simulink model "NONLINEAR_MODEL11"  (R2017b)
settings: Solver=VariableStepAuto  StartTime=0.0  StopTime=50  RelTol=1e-3
values from neighbouring files (symbols this model uses):
  altitude = input('Enter the altitude for the simulation (ft)  :  ')    [FindF16Dynamics.m]    (also in run_me.m = input(' altitude ( 0 ~ 40000 ft ) : '); trim_F16.m = alt)
  control_trim = u0    [find_trim.m]
  state_trim = steady_state( state )    [find_trim.m]
  trim_state = xu(1:12)    [trim_F16.m]
  velocity = input('Enter the velocity for the simulation (ft/s):  ')    [FindF16Dynamics.m]    (also in run_me.m = input(' true velocity ( 350 ~ 1000 ft/sec ) : '); trim_F16.m = vel)
libraries: simulink x7, F16_Actuator_Library x1
settings Model: Creator=monster  LastModifiedBy=monster

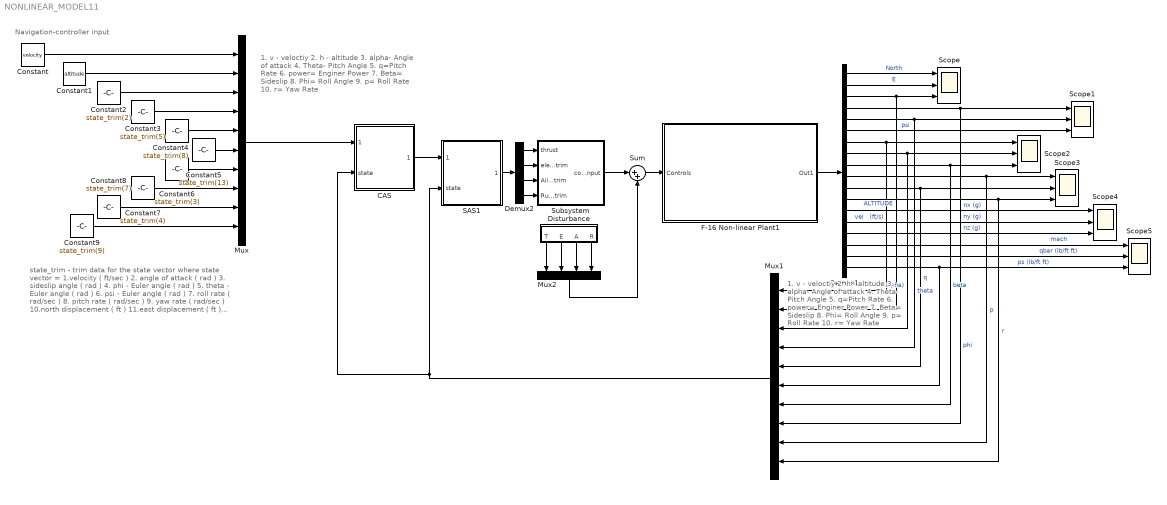
== system NONLINEAR_MODEL11 ==
  note: Navigation-controller input
  note: 1. v - veloctiy
      |
      | 2. h - altitude
      |
      | 3. alpha- Angle of attack
      |
      | 4. Theta- Pitch Angle
      |
      | 5. q=Pitch Rate
      |
      | 6. power= Enginer Power
      |
      | 7. Beta= Sideslip
      |
      | 8. Phi= Roll Angle
      |
      | 9. p= Roll Rate
      |
      | 10. r= Yaw Rate
  note: 1. v - veloctiy
      |
      | 2. h - altitude
      |
      | 3. alpha- Angle of attack
      |
      | 4. Theta- Pitch Angle
      |
      | 5. q=Pitch Rate
      |
      | 6. power= Enginer Power
      |
      | 7. Beta= Sideslip
      |
      | 8. Phi= Roll Angle
      |
      | 9. p= Roll Rate
      |
      | 10. r= Yaw Rate
  note: state_trim   - trim data for the state vector where
      |       state vector =
      | 1.velocity             ( ft/sec )
      | 2. angle of attack      ( rad )
      |  3. sideslip angle       ( rad )
      | 4. phi   - Euler angle  ( rad )
      | 5. theta - Euler angle  ( rad )
      |    6. psi   - Euler angle  ( rad )
      |   7. roll rate            ( rad/sec )
      | 8. pitch rate           ( rad/sec )
      |  9. yaw rate             ( rad/sec )
      | 10.north displacement   ( ft )
      | 11.east displacement    ( ft )
      | 12.altitude             ( ft )
      | 13.power  ( percent, 0 <= pow <= 100 )
  " Disturbance" : Subsystem
  CAS : Subsystem
  Constant : Constant  Value=velocity
  Constant1 : Constant  Value=altitude
  Constant2 : Constant  Value=state_trim(2)
  Constant3 : Constant  Value=state_trim(5)
  Constant4 : Constant  Value=state_trim(8)
  Constant5 : Constant  Value=state_trim(13)
  Constant6 : Constant  Value=state_trim(3)
  Constant7 : Constant  Value=state_trim(4)
  Constant8 : Constant  Value=state_trim(7)
  Constant9 : Constant  Value=state_trim(9)
  Demux1 : Demux  Outputs=18
  Demux2 : Demux
  F-16 Non-linear Plant1 : Subsystem
      mask Display: image('D:\Dropbox\M.eng\fall2017\flight control system\FDC\project\control surface.PNG');
  Mux : Mux  Inputs=10
  Mux1 : Mux  Inputs=10
  Mux2 : Mux
  SAS1 : Subsystem
  Scope{,1..5} (6 alike) : Scope  NumInputPorts=3
  Subsystem : Subsystem
  Sum : Sum  Inputs=|++
  wires:
  Demux1/11 -> Scope3/2, Mux1/5  "q"
  Demux1/18 -> Mux1/6, Scope5/3  "ps (lb/ft ft)"
  Demux1/16 -> Scope5/1  "mach"
  Demux1/17 -> Scope5/2  "qbar (lb/ft ft)"
  F-16 Non-linear Plant1/1(Out1) -> Demux1/1
  Demux1/7 -> Mux1/1, Scope2/1  "vel   (ft/s)"
  Demux1/10 -> Mux1/9, Scope3/1  "p"
  Demux1/9 -> Mux1/7, Scope2/3  "beta"
  Demux1/6 -> Scope1/3  "psi"
  Demux1/14 -> Scope4/2  "ny (g)"
  Demux1/2 -> Scope/2  "E"
  Demux1/12 -> Mux1/10, Scope3/3  "r"
  Demux1/5 -> Mux1/4, Scope1/2  "theta"
  Demux1/15 -> Scope4/3  "nz (g)"
  Demux1/3 -> Mux1/2, Scope/3  "ALTITUDE"
  Demux1/1 -> Scope/1  "North"
  Demux1/8 -> Mux1/3, Scope2/2  "alpha)"
  Demux1/4 -> Mux1/8, Scope1/1  "phi"
  Demux1/13 -> Scope4/1  "nx (g)"
  Constant4/1 -> Mux/5
  " Disturbance"/1(T) -> Mux2/1
  Mux2/1 -> Sum/2
  Constant2/1 -> Mux/3
  Mux1/1 -> CAS/2(state), SAS1/2(state)
  Constant7/1 -> Mux/8
  Constant9/1 -> Mux/10
  Mux/1 -> CAS/1(reference)
  SAS1/1(control_input) -> Demux2/1
  Demux2/4 -> Subsystem/4(Rudder_trim)
  Constant5/1 -> Mux/6
  Constant8/1 -> Mux/9
  Subsystem/1(control_input) -> Sum/1
  Demux2/1 -> Subsystem/1(thrust)
  " Disturbance"/4(R) -> Mux2/4
  Demux2/2 -> Subsystem/2(elevator_trim)
  " Disturbance"/2(E) -> Mux2/2
  Constant6/1 -> Mux/7
  Demux2/3 -> Subsystem/3(Aileron_trim)
  Constant1/1 -> Mux/2
  CAS/1(control_input) -> SAS1/1(reference)
  Constant3/1 -> Mux/4
  Constant/1 -> Mux/1
  " Disturbance"/3(A) -> Mux2/3
  Sum/1 -> F-16 Non-linear Plant1/1(Controls)

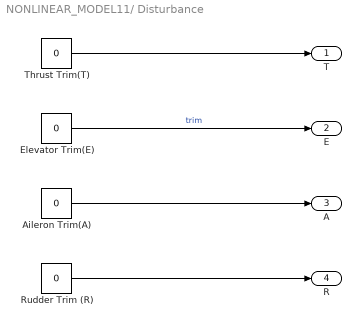
== system NONLINEAR_MODEL11/ Disturbance ==
  "Aileron Trim(A) " : Constant  Value=0
  "Elevator Trim(E) " : Constant  Value=0  VectorParams1D=off
  Rudder Trim (R) : Constant  Value=0
  "Thrust Trim(T) " : Constant  Value=0
  T : Outport
  E : Outport  Port=2
  A : Outport  Port=3
  R : Outport  Port=4
  wires:
  "Aileron Trim(A) "/1 -> A/1
  "Elevator Trim(E) "/1 -> E/1  "trim"
  "Thrust Trim(T) "/1 -> T/1
  Rudder Trim (R)/1 -> R/1

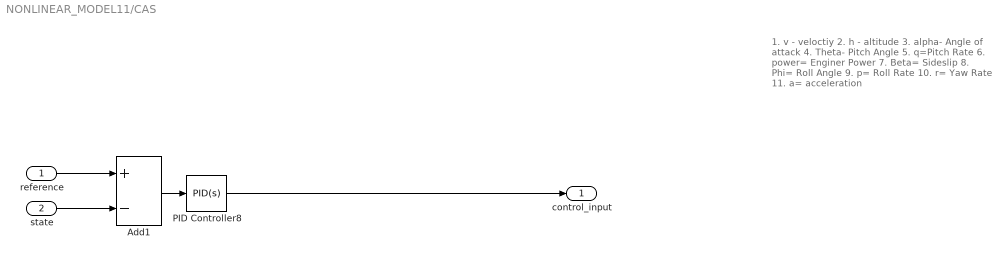
== system NONLINEAR_MODEL11/CAS ==
  note: 1. v - veloctiy
      |
      | 2. h - altitude
      |
      | 3. alpha- Angle of attack
      |
      | 4. Theta- Pitch Angle
      |
      | 5. q=Pitch Rate
      |
      | 6. power= Enginer Power
      |
      | 7. Beta= Sideslip
      |
      | 8. Phi= Roll Angle
      |
      | 9. p= Roll Rate
      |
      | 10. r= Yaw Rate
      |
      | 11. a= acceleration
  reference : Inport
  state : Inport  Port=2
  Add1 : Sum  Inputs=+-
  PID Controller8 : simulink/Continuous/PID Controller  Controller=PID  TimeDomain=Continuous-time  SampleTime=-1  IntegratorMethod=Forward Euler  FilterMethod=Forward Euler  Form=Parallel  UseFilter=on  ControllerParametersSource=internal  P=-49327.5398646116  I=-459229.123376859  D=-1288.80480278299  N=1181.77739704053  InitialConditionSource=internal  InitialConditionForIntegrator=0  InitialConditionForFilter=0  ExternalReset=none  LimitOutput=off  UpperSaturationLimit=inf  LowerSaturationLimit=-inf  LinearizeAsGain=on  AntiWindupMode=none  Kb=1  TrackingMode=off  Kt=1  PParamMin=[]  PParamMax=[]  IParamMin=[]  IParamMax=[]  DParamMin=[]  DParamMax=[]  NParamMin=[]  NParamMax=[]  KbParamMin=[]  KbParamMax=[]  KtParamMin=[]  KtParamMax=[]  POutMin=[]  POutMax=[]  IOutMin=[]  IOutMax=[]  DOutMin=[]  DOutMax=[]  NOutMin=[]  NOutMax=[]  KbOutMin=[]  KbOutMax=[]  KtOutMin=[]  KtOutMax=[]  IntegratorOutMin=[]  IntegratorOutMax=[]  FilterOutMin=[]  FilterOutMax=[]  SumOutMin=[]  SumOutMax=[]  SumI1OutMin=[]  SumI1OutMax=[]  SumI2OutMin=[]  SumI2OutMax=[]  SumI3OutMin=[]  SumI3OutMax=[]  SumDOutMin=[]  SumDOutMax=[]  SaturationOutMin=[]  SaturationOutMax=[]  IntegratorContinuousStateAttributes=''  IntegratorStateMustResolveToSignalObject=off  IntegratorRTWStateStorageClass=Auto  FilterContinuousStateAttributes=''  FilterStateMustResolveToSignalObject=off  FilterRTWStateStorageClass=Auto  DifferentiatorICPrevScaledInput=0  DifferentiatorOutMin=[]  DifferentiatorOutMax=[]  InitialConditionSetting=State (most efficient)  FilterDiffOutCoefMin=[]  FilterDiffOutCoefMax=[]  SumDenOutMin=[]  SumDenOutMax=[]  SumNumOutMin=[]  SumNumOutMax=[]  ReciprocalOutMin=[]  ReciprocalOutMax=[]  DivideOutMin=[]  DivideOutMax=[]  TunerSelectOption=Transfer Function Based (PID Tuner App)
  control_input : Outport
  wires:
  PID Controller8/1 -> control_input/1
  Add1/1 -> PID Controller8/1
  reference/1 -> Add1/1
  state/1 -> Add1/2

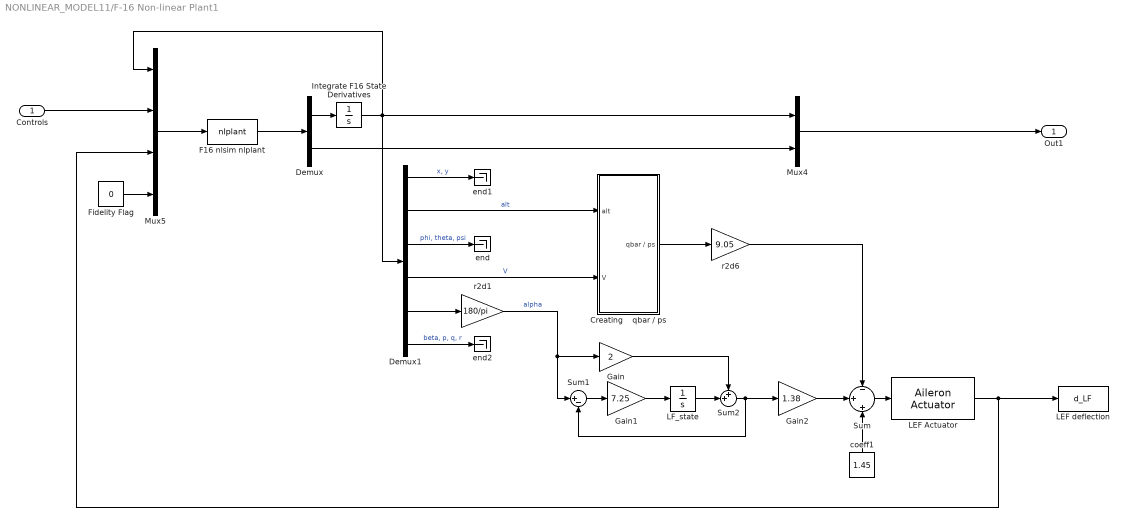
== system NONLINEAR_MODEL11/F-16 Non-linear Plant1 ==
  Controls : Inport
  Creating    qbar / ps : Subsystem
  Demux : Demux  Outputs=[12 6]
  Demux1 : Demux  Outputs=[2,1,3,1,1,4]
  F16 nlsim nlplant : MATLABFcn  MATLABFcn=nlplant  OutputDimensions=18  OutputSignalType=real
  Fidelity Flag : Constant  Value=0
  Gain : Gain  Gain=2  SaturateOnIntegerOverflow=on  OutDataTypeStr=Inherit: Same as input  ParamDataTypeStr=Inherit: Same as input
  Gain1 : Gain  Gain=7.25  SaturateOnIntegerOverflow=on  OutDataTypeStr=Inherit: Same as input  ParamDataTypeStr=Inherit: Same as input
  Gain2 : Gain  Gain=1.38  SaturateOnIntegerOverflow=on  OutDataTypeStr=Inherit: Same as input  ParamDataTypeStr=Inherit: Same as input
  Integrate F16 State Derivatives : Integrator  InitialCondition=[trim_state(1:12)]
  LEF Actuator : F16_Actuator_Library/Aileron Actuator
  LEF deflection : ToWorkspace  VariableName=d_LF  SampleTime=-1
      settings: Decimation=100
  LF_state : Integrator  InitialCondition=-state_trim(8)*180/pi
  Mux4 : Mux  Inputs=2
  Mux5 : Mux  Inputs=[12 4 1 1]
  Sum : Sum  Inputs=-|+|+  SaturateOnIntegerOverflow=on  InputSameDT=on  OutDataTypeStr=Inherit: Same as first input
  Sum1 : Sum  Inputs=|+-  SaturateOnIntegerOverflow=on  InputSameDT=on  OutDataTypeStr=Inherit: Same as first input
  Sum2 : Sum  Inputs=++|  SaturateOnIntegerOverflow=on  InputSameDT=on  OutDataTypeStr=Inherit: Same as first input
  coeff1 : Constant  Value=1.45
  end : Terminator
  end1 : Terminator
  end2 : Terminator
  r2d1 : Gain  Gain=180/pi  SaturateOnIntegerOverflow=on  OutDataTypeStr=Inherit: Same as input  ParamDataTypeStr=Inherit: Same as input
  r2d6 : Gain  Gain=9.05  SaturateOnIntegerOverflow=on  OutDataTypeStr=Inherit: Same as input  ParamDataTypeStr=Inherit: Same as input
  Out1 : Outport
  wires:
  Mux5/1 -> F16 nlsim nlplant/1
  Fidelity Flag/1 -> Mux5/4
  LEF Actuator/1 -> LEF deflection/1, Mux5/3
  Controls/1 -> Mux5/2
  Demux/1 -> Integrate F16 State Derivatives/1
  Demux/2 -> Mux4/2
  Mux4/1 -> Out1/1
  F16 nlsim nlplant/1 -> Demux/1
  Demux1/2 -> Creating    qbar / ps/1(alt)  "alt"
  r2d6/1 -> Sum/1
  Creating    qbar / ps/1(qbar / ps) -> r2d6/1
  Demux1/4 -> Creating    qbar / ps/2(V)  "V"
  r2d1/1 -> Sum1/1, Gain/1  "alpha"
  LF_state/1 -> Sum2/2
  Sum2/1 -> Sum1/2, Gain2/1
  coeff1/1 -> Sum/3
  Demux1/6 -> end2/1  "beta, p, q, r"
  Demux1/5 -> r2d1/1
  Demux1/1 -> end1/1  "x, y"
  Gain2/1 -> Sum/2
  Gain/1 -> Sum2/1
  Gain1/1 -> LF_state/1
  Sum1/1 -> Gain1/1
  Integrate F16 State Derivatives/1 -> Demux1/1, Mux4/1, Mux5/1
  Demux1/3 -> end/1  "phi, theta, psi"
  Sum/1 -> LEF Actuator/1

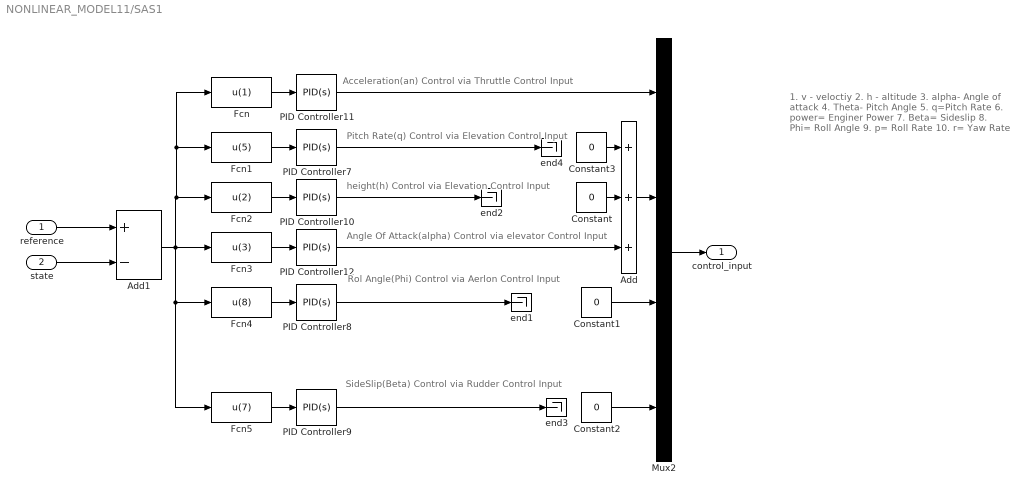
== system NONLINEAR_MODEL11/SAS1 ==
  note: Rol Angle(Phi) Control via Aerlon Control Input
  note: height(h) Control via Elevation Control Input
  note: Pitch Rate(q) Control via Elevation Control Input
  note: Acceleration(an) Control via Thruttle Control Input
  note: Angle Of Attack(alpha) Control via elevator Control Input
  note: SideSlip(Beta) Control via Rudder Control Input
  note: 1. v - veloctiy
      |
      | 2. h - altitude
      |
      | 3. alpha- Angle of attack
      |
      | 4. Theta- Pitch Angle
      |
      | 5. q=Pitch Rate
      |
      | 6. power= Enginer Power
      |
      | 7. Beta= Sideslip
      |
      | 8. Phi= Roll Angle
      |
      | 9. p= Roll Rate
      |
      | 10. r= Yaw Rate
  reference : Inport
  state : Inport  Port=2
  Add : Sum  Inputs=+++
  Add1 : Sum  Inputs=+-
  Constant{,1..3} (4 alike) : Constant  Value=0
  Fcn : Fcn  Expr=u(1)
  Fcn1 : Fcn  Expr=u(5)
  Fcn2 : Fcn  Expr=u(2)
  Fcn3 : Fcn  Expr=u(3)
  Fcn4 : Fcn  Expr=u(8)
  Fcn5 : Fcn  Expr=u(7)
  Mux2 : Mux
  PID Controller10 : simulink/Continuous/PID Controller  Controller=PID  TimeDomain=Continuous-time  SampleTime=-1  IntegratorMethod=Forward Euler  FilterMethod=Forward Euler  Form=Parallel  UseFilter=on  ControllerParametersSource=internal  P=24508600.1259152  I=4501969741.89748  D=28958.3047379278  N=690409.793644926  InitialConditionSource=internal  InitialConditionForIntegrator=0  InitialConditionForFilter=0  ExternalReset=none  LimitOutput=off  UpperSaturationLimit=inf  LowerSaturationLimit=-inf  LinearizeAsGain=on  AntiWindupMode=none  Kb=1  TrackingMode=off  Kt=1  PParamMin=[]  PParamMax=[]  IParamMin=[]  IParamMax=[]  DParamMin=[]  DParamMax=[]  NParamMin=[]  NParamMax=[]  KbParamMin=[]  KbParamMax=[]  KtParamMin=[]  KtParamMax=[]  POutMin=[]  POutMax=[]  IOutMin=[]  IOutMax=[]  DOutMin=[]  DOutMax=[]  NOutMin=[]  NOutMax=[]  KbOutMin=[]  KbOutMax=[]  KtOutMin=[]  KtOutMax=[]  IntegratorOutMin=[]  IntegratorOutMax=[]  FilterOutMin=[]  FilterOutMax=[]  SumOutMin=[]  SumOutMax=[]  SumI1OutMin=[]  SumI1OutMax=[]  SumI2OutMin=[]  SumI2OutMax=[]  SumI3OutMin=[]  SumI3OutMax=[]  SumDOutMin=[]  SumDOutMax=[]  SaturationOutMin=[]  SaturationOutMax=[]  IntegratorContinuousStateAttributes=''  IntegratorStateMustResolveToSignalObject=off  IntegratorRTWStateStorageClass=Auto  FilterContinuousStateAttributes=''  FilterStateMustResolveToSignalObject=off  FilterRTWStateStorageClass=Auto  DifferentiatorICPrevScaledInput=0  DifferentiatorOutMin=[]  DifferentiatorOutMax=[]  InitialConditionSetting=State (most efficient)  FilterDiffOutCoefMin=[]  FilterDiffOutCoefMax=[]  SumDenOutMin=[]  SumDenOutMax=[]  SumNumOutMin=[]  SumNumOutMax=[]  ReciprocalOutMin=[]  ReciprocalOutMax=[]  DivideOutMin=[]  DivideOutMax=[]  TunerSelectOption=Transfer Function Based (PID Tuner App)
  PID Controller11 : simulink/Continuous/PID Controller  Controller=PID  TimeDomain=Continuous-time  SampleTime=-1  IntegratorMethod=Forward Euler  FilterMethod=Forward Euler  Form=Parallel  UseFilter=on  ControllerParametersSource=internal  P=133  I=3928  D=9898  N=109037.560099343  InitialConditionSource=internal  InitialConditionForIntegrator=0  InitialConditionForFilter=0  ExternalReset=none  LimitOutput=off  UpperSaturationLimit=inf  LowerSaturationLimit=-inf  LinearizeAsGain=on  AntiWindupMode=none  Kb=1  TrackingMode=off  Kt=1  PParamMin=[]  PParamMax=[]  IParamMin=[]  IParamMax=[]  DParamMin=[]  DParamMax=[]  NParamMin=[]  NParamMax=[]  KbParamMin=[]  KbParamMax=[]  KtParamMin=[]  KtParamMax=[]  POutMin=[]  POutMax=[]  IOutMin=[]  IOutMax=[]  DOutMin=[]  DOutMax=[]  NOutMin=[]  NOutMax=[]  KbOutMin=[]  KbOutMax=[]  KtOutMin=[]  KtOutMax=[]  IntegratorOutMin=[]  IntegratorOutMax=[]  FilterOutMin=[]  FilterOutMax=[]  SumOutMin=[]  SumOutMax=[]  SumI1OutMin=[]  SumI1OutMax=[]  SumI2OutMin=[]  SumI2OutMax=[]  SumI3OutMin=[]  SumI3OutMax=[]  SumDOutMin=[]  SumDOutMax=[]  SaturationOutMin=[]  SaturationOutMax=[]  IntegratorContinuousStateAttributes=''  IntegratorStateMustResolveToSignalObject=off  IntegratorRTWStateStorageClass=Auto  FilterContinuousStateAttributes=''  FilterStateMustResolveToSignalObject=off  FilterRTWStateStorageClass=Auto  DifferentiatorICPrevScaledInput=0  DifferentiatorOutMin=[]  DifferentiatorOutMax=[]  InitialConditionSetting=State (most efficient)  FilterDiffOutCoefMin=[]  FilterDiffOutCoefMax=[]  SumDenOutMin=[]  SumDenOutMax=[]  SumNumOutMin=[]  SumNumOutMax=[]  ReciprocalOutMin=[]  ReciprocalOutMax=[]  DivideOutMin=[]  DivideOutMax=[]  TunerSelectOption=Transfer Function Based (PID Tuner App)
  PID Controller12 : simulink/Continuous/PID Controller  Controller=PID  TimeDomain=Continuous-time  SampleTime=-1  IntegratorMethod=Forward Euler  FilterMethod=Forward Euler  Form=Parallel  UseFilter=on  ControllerParametersSource=internal  P=-170.14183467408  I=-465.695324804371  D=-13.6839697818054  N=105.697856042613  InitialConditionSource=internal  InitialConditionForIntegrator=0  InitialConditionForFilter=0  ExternalReset=none  LimitOutput=off  UpperSaturationLimit=inf  LowerSaturationLimit=-inf  LinearizeAsGain=on  AntiWindupMode=none  Kb=1  TrackingMode=off  Kt=1  PParamMin=[]  PParamMax=[]  IParamMin=[]  IParamMax=[]  DParamMin=[]  DParamMax=[]  NParamMin=[]  NParamMax=[]  KbParamMin=[]  KbParamMax=[]  KtParamMin=[]  KtParamMax=[]  POutMin=[]  POutMax=[]  IOutMin=[]  IOutMax=[]  DOutMin=[]  DOutMax=[]  NOutMin=[]  NOutMax=[]  KbOutMin=[]  KbOutMax=[]  KtOutMin=[]  KtOutMax=[]  IntegratorOutMin=[]  IntegratorOutMax=[]  FilterOutMin=[]  FilterOutMax=[]  SumOutMin=[]  SumOutMax=[]  SumI1OutMin=[]  SumI1OutMax=[]  SumI2OutMin=[]  SumI2OutMax=[]  SumI3OutMin=[]  SumI3OutMax=[]  SumDOutMin=[]  SumDOutMax=[]  SaturationOutMin=[]  SaturationOutMax=[]  IntegratorContinuousStateAttributes=''  IntegratorStateMustResolveToSignalObject=off  IntegratorRTWStateStorageClass=Auto  FilterContinuousStateAttributes=''  FilterStateMustResolveToSignalObject=off  FilterRTWStateStorageClass=Auto  DifferentiatorICPrevScaledInput=0  DifferentiatorOutMin=[]  DifferentiatorOutMax=[]  InitialConditionSetting=State (most efficient)  FilterDiffOutCoefMin=[]  FilterDiffOutCoefMax=[]  SumDenOutMin=[]  SumDenOutMax=[]  SumNumOutMin=[]  SumNumOutMax=[]  ReciprocalOutMin=[]  ReciprocalOutMax=[]  DivideOutMin=[]  DivideOutMax=[]  TunerSelectOption=Transfer Function Based (PID Tuner App)
  PID Controller7 : simulink/Continuous/PID Controller  Controller=PID  TimeDomain=Continuous-time  SampleTime=-1  IntegratorMethod=Forward Euler  FilterMethod=Forward Euler  Form=Parallel  UseFilter=on  ControllerParametersSource=internal  P=-2409.99420452658  I=-41171.6281036838  D=-4.63151383685818  N=352.425457454863  InitialConditionSource=internal  InitialConditionForIntegrator=0  InitialConditionForFilter=0  ExternalReset=none  LimitOutput=off  UpperSaturationLimit=inf  LowerSaturationLimit=-inf  LinearizeAsGain=on  AntiWindupMode=none  Kb=1  TrackingMode=off  Kt=1  PParamMin=[]  PParamMax=[]  IParamMin=[]  IParamMax=[]  DParamMin=[]  DParamMax=[]  NParamMin=[]  NParamMax=[]  KbParamMin=[]  KbParamMax=[]  KtParamMin=[]  KtParamMax=[]  POutMin=[]  POutMax=[]  IOutMin=[]  IOutMax=[]  DOutMin=[]  DOutMax=[]  NOutMin=[]  NOutMax=[]  KbOutMin=[]  KbOutMax=[]  KtOutMin=[]  KtOutMax=[]  IntegratorOutMin=[]  IntegratorOutMax=[]  FilterOutMin=[]  FilterOutMax=[]  SumOutMin=[]  SumOutMax=[]  SumI1OutMin=[]  SumI1OutMax=[]  SumI2OutMin=[]  SumI2OutMax=[]  SumI3OutMin=[]  SumI3OutMax=[]  SumDOutMin=[]  SumDOutMax=[]  SaturationOutMin=[]  SaturationOutMax=[]  IntegratorContinuousStateAttributes=''  IntegratorStateMustResolveToSignalObject=off  IntegratorRTWStateStorageClass=Auto  FilterContinuousStateAttributes=''  FilterStateMustResolveToSignalObject=off  FilterRTWStateStorageClass=Auto  DifferentiatorICPrevScaledInput=0  DifferentiatorOutMin=[]  DifferentiatorOutMax=[]  InitialConditionSetting=State (most efficient)  FilterDiffOutCoefMin=[]  FilterDiffOutCoefMax=[]  SumDenOutMin=[]  SumDenOutMax=[]  SumNumOutMin=[]  SumNumOutMax=[]  ReciprocalOutMin=[]  ReciprocalOutMax=[]  DivideOutMin=[]  DivideOutMax=[]  TunerSelectOption=Transfer Function Based (PID Tuner App)
  PID Controller8 : simulink/Continuous/PID Controller  Controller=PID  TimeDomain=Continuous-time  SampleTime=-1  IntegratorMethod=Forward Euler  FilterMethod=Forward Euler  Form=Parallel  UseFilter=on  ControllerParametersSource=internal  P=-49327.5398646116  I=-459229.123376859  D=-1288.80480278299  N=1181.77739704053  InitialConditionSource=internal  InitialConditionForIntegrator=0  InitialConditionForFilter=0  ExternalReset=none  LimitOutput=off  UpperSaturationLimit=inf  LowerSaturationLimit=-inf  LinearizeAsGain=on  AntiWindupMode=none  Kb=1  TrackingMode=off  Kt=1  PParamMin=[]  PParamMax=[]  IParamMin=[]  IParamMax=[]  DParamMin=[]  DParamMax=[]  NParamMin=[]  NParamMax=[]  KbParamMin=[]  KbParamMax=[]  KtParamMin=[]  KtParamMax=[]  POutMin=[]  POutMax=[]  IOutMin=[]  IOutMax=[]  DOutMin=[]  DOutMax=[]  NOutMin=[]  NOutMax=[]  KbOutMin=[]  KbOutMax=[]  KtOutMin=[]  KtOutMax=[]  IntegratorOutMin=[]  IntegratorOutMax=[]  FilterOutMin=[]  FilterOutMax=[]  SumOutMin=[]  SumOutMax=[]  SumI1OutMin=[]  SumI1OutMax=[]  SumI2OutMin=[]  SumI2OutMax=[]  SumI3OutMin=[]  SumI3OutMax=[]  SumDOutMin=[]  SumDOutMax=[]  SaturationOutMin=[]  SaturationOutMax=[]  IntegratorContinuousStateAttributes=''  IntegratorStateMustResolveToSignalObject=off  IntegratorRTWStateStorageClass=Auto  FilterContinuousStateAttributes=''  FilterStateMustResolveToSignalObject=off  FilterRTWStateStorageClass=Auto  DifferentiatorICPrevScaledInput=0  DifferentiatorOutMin=[]  DifferentiatorOutMax=[]  InitialConditionSetting=State (most efficient)  FilterDiffOutCoefMin=[]  FilterDiffOutCoefMax=[]  SumDenOutMin=[]  SumDenOutMax=[]  SumNumOutMin=[]  SumNumOutMax=[]  ReciprocalOutMin=[]  ReciprocalOutMax=[]  DivideOutMin=[]  DivideOutMax=[]  TunerSelectOption=Transfer Function Based (PID Tuner App)
  PID Controller9 : simulink/Continuous/PID Controller  Controller=PID  TimeDomain=Continuous-time  SampleTime=-1  IntegratorMethod=Forward Euler  FilterMethod=Forward Euler  Form=Parallel  UseFilter=on  ControllerParametersSource=internal  P=908.491475757153  I=143.160579860217  D=1280.97081759687  N=3086.89831654681  InitialConditionSource=internal  InitialConditionForIntegrator=0  InitialConditionForFilter=0  ExternalReset=none  LimitOutput=off  UpperSaturationLimit=inf  LowerSaturationLimit=-inf  LinearizeAsGain=on  AntiWindupMode=none  Kb=1  TrackingMode=off  Kt=1  PParamMin=[]  PParamMax=[]  IParamMin=[]  IParamMax=[]  DParamMin=[]  DParamMax=[]  NParamMin=[]  NParamMax=[]  KbParamMin=[]  KbParamMax=[]  KtParamMin=[]  KtParamMax=[]  POutMin=[]  POutMax=[]  IOutMin=[]  IOutMax=[]  DOutMin=[]  DOutMax=[]  NOutMin=[]  NOutMax=[]  KbOutMin=[]  KbOutMax=[]  KtOutMin=[]  KtOutMax=[]  IntegratorOutMin=[]  IntegratorOutMax=[]  FilterOutMin=[]  FilterOutMax=[]  SumOutMin=[]  SumOutMax=[]  SumI1OutMin=[]  SumI1OutMax=[]  SumI2OutMin=[]  SumI2OutMax=[]  SumI3OutMin=[]  SumI3OutMax=[]  SumDOutMin=[]  SumDOutMax=[]  SaturationOutMin=[]  SaturationOutMax=[]  IntegratorContinuousStateAttributes=''  IntegratorStateMustResolveToSignalObject=off  IntegratorRTWStateStorageClass=Auto  FilterContinuousStateAttributes=''  FilterStateMustResolveToSignalObject=off  FilterRTWStateStorageClass=Auto  DifferentiatorICPrevScaledInput=0  DifferentiatorOutMin=[]  DifferentiatorOutMax=[]  InitialConditionSetting=State (most efficient)  FilterDiffOutCoefMin=[]  FilterDiffOutCoefMax=[]  SumDenOutMin=[]  SumDenOutMax=[]  SumNumOutMin=[]  SumNumOutMax=[]  ReciprocalOutMin=[]  ReciprocalOutMax=[]  DivideOutMin=[]  DivideOutMax=[]  TunerSelectOption=Transfer Function Based (PID Tuner App)
  end{1..4} (4 alike) : Terminator
  control_input : Outport
  wires:
  Mux2/1 -> control_input/1
  PID Controller11/1 -> Mux2/1
  Fcn5/1 -> PID Controller9/1
  Fcn3/1 -> PID Controller12/1
  PID Controller7/1 -> end4/1
  Fcn2/1 -> PID Controller10/1
  Fcn1/1 -> PID Controller7/1
  PID Controller8/1 -> end1/1
  Fcn4/1 -> PID Controller8/1
  Fcn/1 -> PID Controller11/1
  PID Controller10/1 -> end2/1
  Add/1 -> Mux2/2
  PID Controller12/1 -> Add/3
  PID Controller9/1 -> end3/1
  reference/1 -> Add1/1
  state/1 -> Add1/2
  Add1/1 -> Fcn2/1, Fcn1/1, Fcn/1, Fcn5/1, Fcn4/1, Fcn3/1
  Constant/1 -> Add/2
  Constant1/1 -> Mux2/3
  Constant2/1 -> Mux2/4
  Constant3/1 -> Add/1

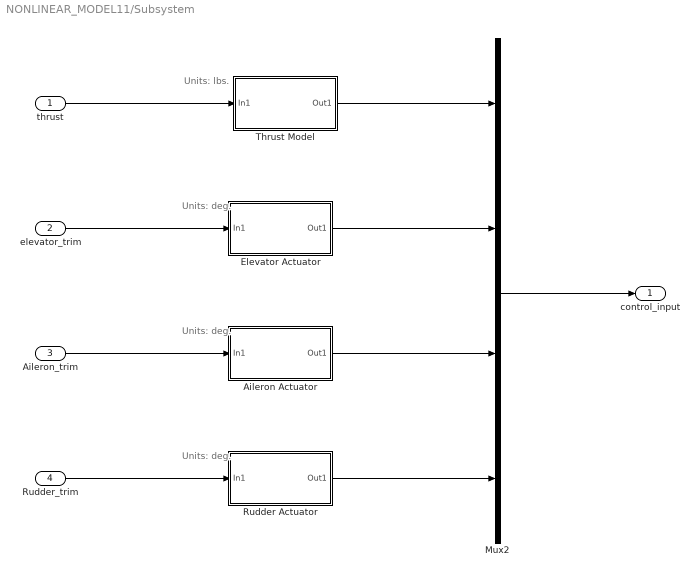
== system NONLINEAR_MODEL11/Subsystem ==
  note: Units: deg.
  note: Units: deg.
  note: Units: lbs.
  note: Units: deg.
  thrust : Inport
  elevator_trim : Inport  Port=2
  Aileron_trim : Inport  Port=3
  Rudder_trim : Inport  Port=4
  Aileron Actuator : Subsystem  AncestorBlock=F16_Actuator_Library/Aileron Actuator
  Elevator Actuator : Subsystem  AncestorBlock=F16_Actuator_Library/Elevator Actuator
  Mux2 : Mux
  Rudder Actuator : Subsystem  AncestorBlock=F16_Actuator_Library/Rudder Actuator
  Thrust Model : Subsystem  AncestorBlock=F16_Actuator_Library/Thrust Model
  control_input : Outport
  wires:
  thrust/1 -> Thrust Model/1(In1)
  Aileron Actuator/1(Out1) -> Mux2/3
  Rudder_trim/1 -> Rudder Actuator/1(In1)
  Elevator Actuator/1(Out1) -> Mux2/2
  Rudder Actuator/1(Out1) -> Mux2/4
  elevator_trim/1 -> Elevator Actuator/1(In1)
  Aileron_trim/1 -> Aileron Actuator/1(In1)
  Thrust Model/1(Out1) -> Mux2/1
  Mux2/1 -> control_input/1

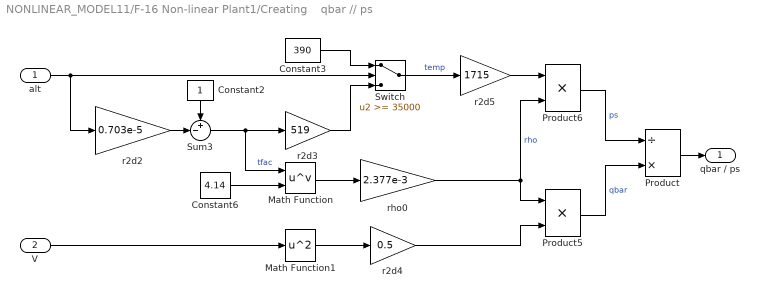
== system NONLINEAR_MODEL11/F-16 Non-linear Plant1/Creating    qbar // ps ==
  alt : Inport
  V : Inport  Port=2
  Constant2 : Constant
  Constant3 : Constant  Value=390
  Constant6 : Constant  Value=4.14
  Math Function : Math  Operator=pow  SaturateOnIntegerOverflow=on
  Math Function1 : Math  Operator=square  SaturateOnIntegerOverflow=on
  Product : Product  Inputs=/*  SaturateOnIntegerOverflow=on  InputSameDT=on  OutDataTypeStr=Inherit: Same as first input
  Product5 : Product  Inputs=**  SaturateOnIntegerOverflow=on  InputSameDT=on  OutDataTypeStr=Inherit: Same as first input
  Product6 : Product  Inputs=**  SaturateOnIntegerOverflow=on  InputSameDT=on  OutDataTypeStr=Inherit: Same as first input
  Sum3 : Sum  Inputs=+-|  SaturateOnIntegerOverflow=on  InputSameDT=on  OutDataTypeStr=Inherit: Same as first input
  Switch : Switch  Threshold=35000  SaturateOnIntegerOverflow=on  InputSameDT=on
  r2d2 : Gain  Gain=0.703e-5  SaturateOnIntegerOverflow=on  OutDataTypeStr=Inherit: Same as input  ParamDataTypeStr=Inherit: Same as input
  r2d3 : Gain  Gain=519  SaturateOnIntegerOverflow=on  OutDataTypeStr=Inherit: Same as input  ParamDataTypeStr=Inherit: Same as input
  r2d4 : Gain  Gain=0.5  SaturateOnIntegerOverflow=on  OutDataTypeStr=Inherit: Same as input  ParamDataTypeStr=Inherit: Same as input
  r2d5 : Gain  Gain=1715  SaturateOnIntegerOverflow=on  OutDataTypeStr=Inherit: Same as input  ParamDataTypeStr=Inherit: Same as input
  rho0 : Gain  Gain=2.377e-3  SaturateOnIntegerOverflow=on  OutDataTypeStr=Inherit: Same as input  ParamDataTypeStr=Inherit: Same as input
  qbar / ps : Outport
  wires:
  alt/1 -> r2d2/1, Switch/2
  Sum3/1 -> Math Function/1, r2d3/1  "tfac"
  Constant3/1 -> Switch/1
  r2d3/1 -> Switch/3
  Constant6/1 -> Math Function/2
  rho0/1 -> Product5/1, Product6/2  "rho"
  Math Function1/1 -> r2d4/1
  r2d2/1 -> Sum3/2
  Constant2/1 -> Sum3/1
  Math Function/1 -> rho0/1
  r2d4/1 -> Product5/2
  Switch/1 -> r2d5/1  "temp"
  r2d5/1 -> Product6/1
  Product6/1 -> Product/1  "ps"
  Product5/1 -> Product/2  "qbar"
  Product/1 -> qbar / ps/1
  V/1 -> Math Function1/1

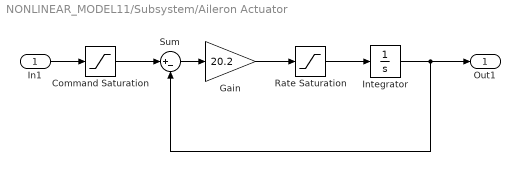
== system NONLINEAR_MODEL11/Subsystem/Aileron Actuator ==
  In1 : Inport
  Command Saturation : Saturate  UpperLimit=21.5  LowerLimit=-21.5
  Gain : Gain  Gain=20.2  SaturateOnIntegerOverflow=on  OutDataTypeStr=Inherit: Same as input  ParamDataTypeStr=Inherit: Same as input
  "Integrator " : Integrator  InitialCondition=control_trim(2)  UpperSaturationLimit=21.5  LowerSaturationLimit=-21.5
  Rate Saturation : Saturate  UpperLimit=80  LowerLimit=-80
  Sum : Sum  Inputs=|+-  SaturateOnIntegerOverflow=on  InputSameDT=on  OutDataTypeStr=Inherit: Same as first input
  Out1 : Outport
  wires:
  "Integrator "/1 -> Sum/2, Out1/1
  Rate Saturation/1 -> "Integrator "/1
  Gain/1 -> Rate Saturation/1
  Sum/1 -> Gain/1
  Command Saturation/1 -> Sum/1
  In1/1 -> Command Saturation/1

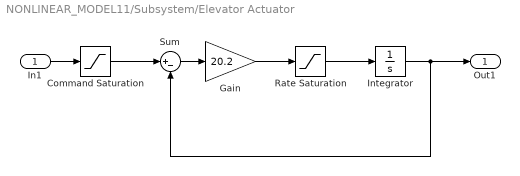
== system NONLINEAR_MODEL11/Subsystem/Elevator Actuator ==
  In1 : Inport
  Command Saturation : Saturate  UpperLimit=25  LowerLimit=-25
  Gain : Gain  Gain=20.2  SaturateOnIntegerOverflow=on  OutDataTypeStr=Inherit: Same as input  ParamDataTypeStr=Inherit: Same as input
  "Integrator " : Integrator  InitialCondition=control_trim(2)  UpperSaturationLimit=25  LowerSaturationLimit=-25
  Rate Saturation : Saturate  UpperLimit=60  LowerLimit=-60
  Sum : Sum  Inputs=|+-  SaturateOnIntegerOverflow=on  InputSameDT=on  OutDataTypeStr=Inherit: Same as first input
  Out1 : Outport
  wires:
  "Integrator "/1 -> Sum/2, Out1/1
  Rate Saturation/1 -> "Integrator "/1
  Gain/1 -> Rate Saturation/1
  Sum/1 -> Gain/1
  Command Saturation/1 -> Sum/1
  In1/1 -> Command Saturation/1

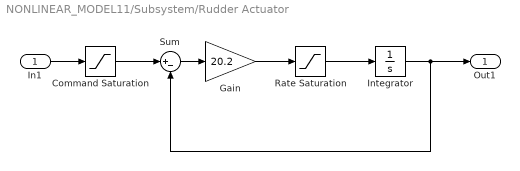
== system NONLINEAR_MODEL11/Subsystem/Rudder Actuator ==
  In1 : Inport
  Command Saturation : Saturate  UpperLimit=30  LowerLimit=-30
  Gain : Gain  Gain=20.2  SaturateOnIntegerOverflow=on  OutDataTypeStr=Inherit: Same as input  ParamDataTypeStr=Inherit: Same as input
  "Integrator " : Integrator  InitialCondition=control_trim(2)  UpperSaturationLimit=30  LowerSaturationLimit=-30
  Rate Saturation : Saturate  UpperLimit=120  LowerLimit=-120
  Sum : Sum  Inputs=|+-  SaturateOnIntegerOverflow=on  InputSameDT=on  OutDataTypeStr=Inherit: Same as first input
  Out1 : Outport
  wires:
  "Integrator "/1 -> Sum/2, Out1/1
  Rate Saturation/1 -> "Integrator "/1
  Gain/1 -> Rate Saturation/1
  Sum/1 -> Gain/1
  Command Saturation/1 -> Sum/1
  In1/1 -> Command Saturation/1

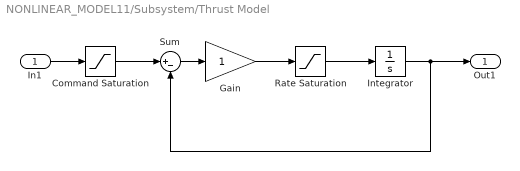
== system NONLINEAR_MODEL11/Subsystem/Thrust Model ==
  In1 : Inport
  Command Saturation : Saturate  UpperLimit=19000  LowerLimit=1000
  Gain : Gain  SaturateOnIntegerOverflow=on  OutDataTypeStr=Inherit: Same as input  ParamDataTypeStr=Inherit: Same as input
  "Integrator " : Integrator  InitialCondition=control_trim(1)  UpperSaturationLimit=30  LowerSaturationLimit=-30
  Rate Saturation : Saturate  UpperLimit=19000  LowerLimit=1000
  Sum : Sum  Inputs=|+-  SaturateOnIntegerOverflow=on  InputSameDT=on  OutDataTypeStr=Inherit: Same as first input
  Out1 : Outport
  wires:
  "Integrator "/1 -> Sum/2, Out1/1
  Rate Saturation/1 -> "Integrator "/1
  Gain/1 -> Rate Saturation/1
  Sum/1 -> Gain/1
  Command Saturation/1 -> Sum/1
  In1/1 -> Command Saturation/1
